simulink model "motor_control_current"  (R2019b)
settings: Solver=VariableStepAuto  StartTime=0.0  StopTime=0.1  RelTol=1e-3
undefined symbols (not defined in the file): Bnew, Gear_Ratio, Jnew, Ke, Ki_current, Kp_current, Kt, La, Ra, Va
settings Model: Creator=이종수  LastModifiedBy=이종수

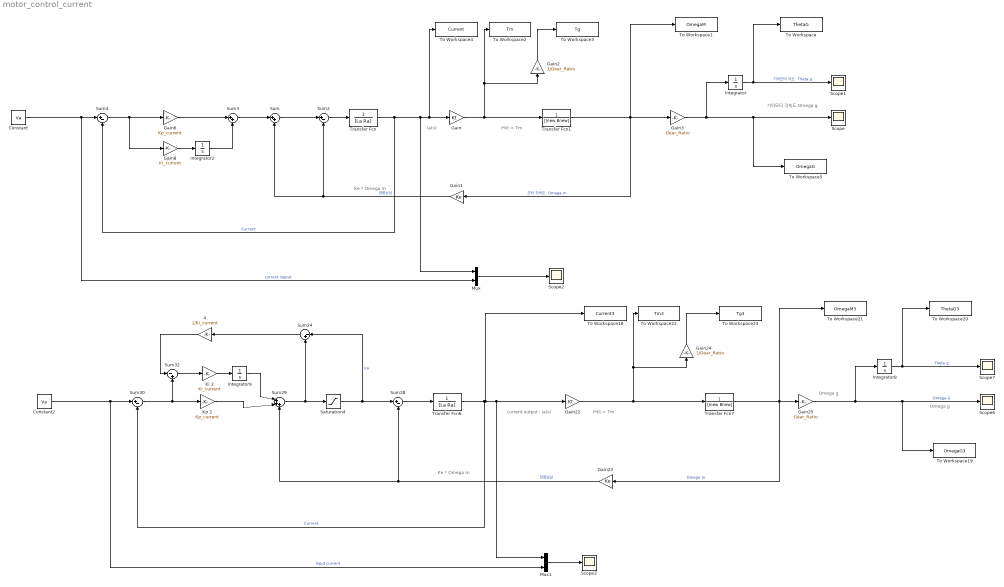
== system motor_control_current ==
  note: I*Kt = Tm
  note: 기어모터 각속도
      | Omega g
  note: Ke * Omega m
  note: Ia(s)
  note: current output : Ia(s)
  note: I*Kt = Tm
  note: Omega g
  note: Ke * Omega m
  note: Omega g
  " 4" : Gain  Gain=1/Ki_current
  Constant : Constant  Value=Va
  Constant2 : Constant  Value=Va
  Gain : Gain  Gain=Kt
  Gain1 : Gain  Gain=Ke
  Gain2 : Gain  Gain=1/Gear_Ratio
  Gain22 : Gain  Gain=Kt
  Gain23 : Gain  Gain=Ke
  Gain24 : Gain  Gain=1/Gear_Ratio
  Gain25 : Gain  Gain=Gear_Ratio
  Gain3 : Gain  Gain=Gear_Ratio
  Gain6 : Gain  Gain=Kp_current
  Gain8 : Gain  Gain=Ki_current
  Integrator{,2,8..9} (4 alike) : Integrator
  Ki 2 : Gain  Gain=Ki_current
  Kp 2 : Gain  Gain=Kp_current
  Mux : Mux  Inputs=2
  Mux1 : Mux  Inputs=2
  Saturation4 : Saturate  UpperLimit=48  LowerLimit=-48
  Scope{,1..3,6..7} (6 alike) : Scope
  Sum : Sum  Inputs=|++
  Sum{2,4,28,30} (4 alike) : Sum  Inputs=|+-
  Sum24 : Sum  Inputs=|-+
  Sum29 : Sum  Inputs=|+++
  Sum3 : Sum  Inputs=|++
  Sum32 : Sum  Inputs=|-+
  To Workspace : ToWorkspace  VariableName=ThetaG  SaveFormat=Structure With Time  SampleTime=-1
  To Workspace1 : ToWorkspace  VariableName=OmegaM  SaveFormat=Structure With Time  SampleTime=-1
  To Workspace18 : ToWorkspace  VariableName=Current3  SaveFormat=Structure With Time  SampleTime=-1
  To Workspace19 : ToWorkspace  VariableName=OmegaG3  SaveFormat=Structure With Time  SampleTime=-1
  To Workspace2 : ToWorkspace  VariableName=Tm  SaveFormat=Structure With Time  SampleTime=-1
  To Workspace20 : ToWorkspace  VariableName=ThetaG3  SaveFormat=Structure With Time  SampleTime=-1
  To Workspace21 : ToWorkspace  VariableName=OmegaM3  SaveFormat=Structure With Time  SampleTime=-1
  To Workspace22 : ToWorkspace  VariableName=Tm3  SaveFormat=Structure With Time  SampleTime=-1
  To Workspace23 : ToWorkspace  VariableName=Tg3  SaveFormat=Structure With Time  SampleTime=-1
  To Workspace3 : ToWorkspace  VariableName=Tg  SaveFormat=Structure With Time  SampleTime=-1
  To Workspace4 : ToWorkspace  VariableName=Current  SaveFormat=Structure With Time  SampleTime=-1
  To Workspace5 : ToWorkspace  VariableName=OmegaG  SaveFormat=Structure With Time  SampleTime=-1
  Transfer Fcn : TransferFcn  Denominator=[La Ra]
  Transfer Fcn1 : TransferFcn  Denominator=[Jnew Bnew]
  Transfer Fcn6 : TransferFcn  Denominator=[La Ra]
  Transfer Fcn7 : TransferFcn  Denominator=[Jnew Bnew]
  wires:
  Transfer Fcn/1 -> Mux/1, To Workspace4/1, Gain/1, Sum4/2  "Current"
  Integrator/1 -> To Workspace/1, Scope1/1  "기어모터 각도  Theta g"
  Transfer Fcn1/1 -> To Workspace1/1, Gain1/1, Gain3/1  "모터 각속도  Omega m"
  Gain/1 -> Gain2/1, To Workspace2/1, Transfer Fcn1/1
  Gain1/1 -> Sum2/2, Sum/2  "전향보상"
  Gain2/1 -> To Workspace3/1
  Gain3/1 -> To Workspace5/1, Scope/1, Integrator/1
  Sum2/1 -> Transfer Fcn/1
  Gain8/1 -> Integrator2/1
  Integrator2/1 -> Sum3/2
  Gain6/1 -> Sum3/1
  Sum/1 -> Sum2/1
  Sum3/1 -> Sum/1
  Constant/1 -> Mux/2, Sum4/1  "current inpput"
  Sum4/1 -> Gain8/1, Gain6/1
  Integrator9/1 -> Sum29/1
  Gain24/1 -> To Workspace23/1
  Transfer Fcn7/1 -> To Workspace21/1, Gain23/1, Gain25/1  "Omega m"
  Sum30/1 -> Kp 2/1, Sum32/2
  Ki 2/1 -> Integrator9/1
  Sum29/1 -> Sum24/2, Saturation4/1
  Transfer Fcn6/1 -> Mux1/1, Gain22/1, To Workspace18/1, Sum30/2  "Current"
  Gain22/1 -> Transfer Fcn7/1, Gain24/1, To Workspace22/1
  Gain23/1 -> Sum29/3, Sum28/2  "전향보상"
  Integrator8/1 -> To Workspace20/1, Scope7/1  "Theta g"
  Saturation4/1 -> Sum24/1, Sum28/1  "Va"
  Sum28/1 -> Transfer Fcn6/1
  " 4"/1 -> Sum32/1
  Kp 2/1 -> Sum29/2
  Gain25/1 -> To Workspace19/1, Scope6/1, Integrator8/1  "Omega G"
  Sum24/1 -> " 4"/1
  Sum32/1 -> Ki 2/1
  Constant2/1 -> Mux1/2, Sum30/1  "Input current"
  Mux/1 -> Scope2/1
  Mux1/1 -> Scope3/1
